simulink model "PathNavHardwareV2"  (R2021a)
settings: Solver=FixedStepAuto  StartTime=0.0  StopTime=10.0  RelTol=1e-3
values from neighbouring files (symbols this model uses):
  axleLength = 0.136    [robotParameters.m]
  ticksPerRot = 20    [robotParameters.m]
  wheelR = 0.031    [robotParameters.m]
undefined symbols (not defined in the file or in its folder): InputPWM, WheelSpeed
libraries: arduinolib x11, pid_lib x5, spsEdgeDetectorLib x2, simulink_extras x1, mobileRoboticsTrainingLib x1
settings Model: SILPILModeSetting=veronly  ExtModeTrigDuration=2  Creator=Marc  LastModifiedBy=Marc
settings OptimizationCC: EnhancedBackFolding=on  PassReuseOutputArgsAs=Individual arguments  ZeroExternalMemoryAtStartup=off  ZeroInternalMemoryAtStartup=off  MaxStackSize=64  OptimizeBlockOrder=speed  DifferentSizesBufferReuse=on  OptimizationCustomize=off  EfficientTunableParamExpr=on
settings DebuggingCC: ParameterTunabilityLossMsg=error
settings HardwareCC: ProdBitPerInt=16  ProdBitPerPointer=16  ProdBitPerSizeT=16  ProdBitPerPtrDiffT=16  ProdLargestAtomicFloat=None  ProdWordSize=8  ProdHWDeviceType=Atmel->AVR  UseEmbeddedCoderFeatures=off  UseSimulinkCoderFeatures=off
settings SFSimCC: MATLABDynamicMemAlloc=off
settings RTWCC: SystemTargetFile=ert.tlc  HardwareBoard=Arduino Leonardo  TemplateMakefile=ert_default_tmf  Toolchain=Arduino AVR
settings CodeAppCC: ForceParamTrailComments=on  IgnoreCustomStorageClasses=off  OperatorAnnotations=on  SimulinkDataObjDesc=on  SFDataObjDesc=on  InsertBlockDesc=on
settings ERTTargetCC: SupportContinuousTime=on  SupportNonInlinedSFcns=on  SupportVariableSizeSignals=on  ExtModeTransport=5  ExtModeStaticAllocSize=250  ExtModeMexFile=ext_serial_win32_comm_leonardo

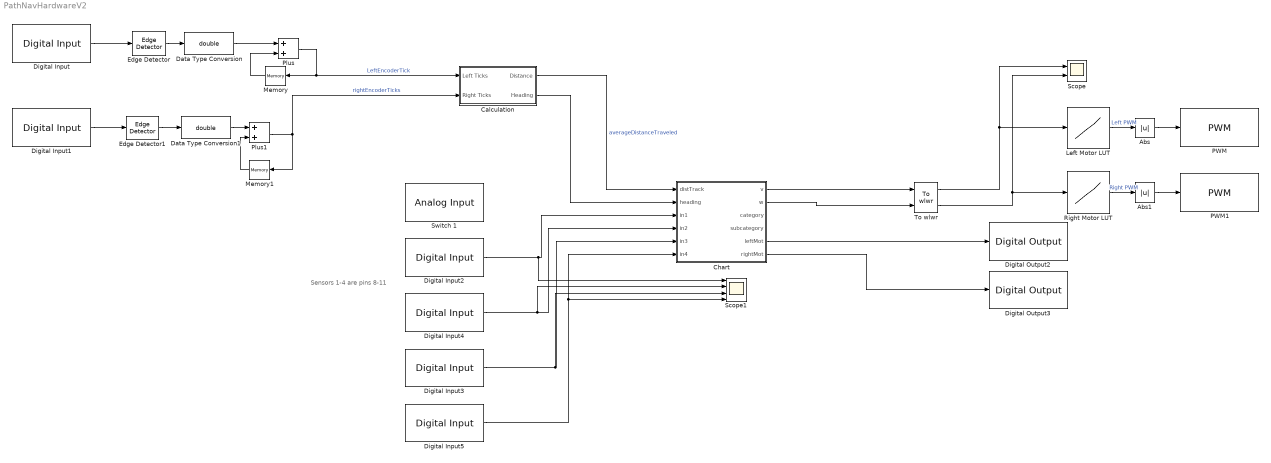
== system PathNavHardwareV2 ==
  note: Sensors 1-4 are pins 8-11
  Abs : Abs
  Abs1 : Abs
  Calculation : Subsystem
  Chart : Stateflow chart  TreatAsAtomicUnit=on
  Data Type Conversion : DataTypeConversion  OutDataTypeStr=double
  Data Type Conversion1 : DataTypeConversion  OutDataTypeStr=double
  Digital Input : arduinolib/Digital Input  pinNumber=2  mode=Default  Direction=input  SampleTime=0.01  blockPlatform=arduino
  Digital Input1 : arduinolib/Digital Input  pinNumber=3  mode=Default  Direction=input  SampleTime=0.01  blockPlatform=arduino
  Digital Input2 : arduinolib/Digital Input  pinNumber=8  mode=Default  Direction=input  SampleTime=0.01  blockPlatform=arduino
  Digital Input3 : arduinolib/Digital Input  pinNumber=10  mode=Default  Direction=input  SampleTime=0.01  blockPlatform=arduino
  Digital Input4 : arduinolib/Digital Input  pinNumber=9  mode=Default  Direction=input  SampleTime=0.01  blockPlatform=arduino
  Digital Input5 : arduinolib/Digital Input  pinNumber=11  mode=Default  Direction=input  SampleTime=0.01  blockPlatform=arduino
  Digital Output2 : arduinolib/Digital Output  pinNumber=4  Direction=output  blockPlatform=arduino
  Digital Output3 : arduinolib/Digital Output  pinNumber=7  Direction=output  blockPlatform=arduino
  Edge Detector : spsEdgeDetectorLib/Edge Detector  model=Either  ic=0  Ts=0
      settings: SourceProductBaseCode=PS
  Edge Detector1 : spsEdgeDetectorLib/Edge Detector  model=Either  ic=0  Ts=0
      settings: SourceProductBaseCode=PS
  Left Motor LUT : Lookup_n-D  NumberOfTableDimensions=1  BreakpointsForDimension1=WheelSpeed  Table=InputPWM  InterpMethod=Nearest  ExtrapMethod=Clip  InternalRulePriority=Speed  RndMeth=Simplest  InputSameDT=on
  Memory : Memory
  Memory1 : Memory
  PWM : arduinolib/PWM  pinNumber=5  frequencyType=Default  desiredFrequency=490.2  achievableFrequency=490.2
  PWM1 : arduinolib/PWM  pinNumber=6  frequencyType=Default  desiredFrequency=490.2  achievableFrequency=490.2
  Plus : Sum
  Plus1 : Sum
  Right Motor LUT : Lookup_n-D  NumberOfTableDimensions=1  BreakpointsForDimension1=WheelSpeed  Table=InputPWM  InterpMethod=Nearest  ExtrapMethod=Clip  InternalRulePriority=Speed  RndMeth=Simplest  InputSameDT=on
  Scope : Scope  NumInputPorts=2
  Scope1 : Scope  NumInputPorts=4
  Switch 1 : arduinolib/Analog Input  pinNumber=0  ReadResultsOnly=off  ConversionTriggerSource=Software  ExternalTriggerType=uint32( 0 )  OutputDataType=uint16  EnableConversionCompleteNotify=off  EnableOuputStatus=off  SampleTime=0.01  blockPlatform=arduino
  To wlwr : mobileRoboticsTrainingLib/To wlwr  axleLength=0.1  wheelR=0.05
  wires:
  Edge Detector1/1 -> Data Type Conversion1/1
  Edge Detector/1 -> Data Type Conversion/1
  Plus1/1 -> Calculation/2(Right Ticks), Memory1/1  "rightEncoderTicks"
  To wlwr/1 -> Scope/1, Left Motor LUT/1
  Digital Input1/1 -> Edge Detector1/1
  Left Motor LUT/1 -> Abs/1  "Left PWM"
  Data Type Conversion/1 -> Plus/1
  Plus/1 -> Calculation/1(Left Ticks), Memory/1  "LeftEncoderTick"
  Digital Input/1 -> Edge Detector/1
  Memory/1 -> Plus/2
  Memory1/1 -> Plus1/2
  Data Type Conversion1/1 -> Plus1/1
  Right Motor LUT/1 -> Abs1/1  "Right PWM"
  To wlwr/2 -> Scope/2, Right Motor LUT/1
  Calculation/1(Distance) -> Chart/1(distTrack)  "averageDistanceTraveled"
  Calculation/2(Heading) -> Chart/2(heading)
  Digital Input2/1 -> Scope1/1, Chart/3(in1)
  Digital Input4/1 -> Scope1/2, Chart/4(in2)
  Digital Input3/1 -> Chart/5(in3), Scope1/3
  Digital Input5/1 -> Scope1/4, Chart/6(in4)
  Chart/1(v) -> To wlwr/1
  Chart/2(w) -> To wlwr/2
  Chart/5(leftMot) -> Digital Output2/1
  Chart/6(rightMot) -> Digital Output3/1
  Abs/1 -> PWM/1
  Abs1/1 -> PWM1/1

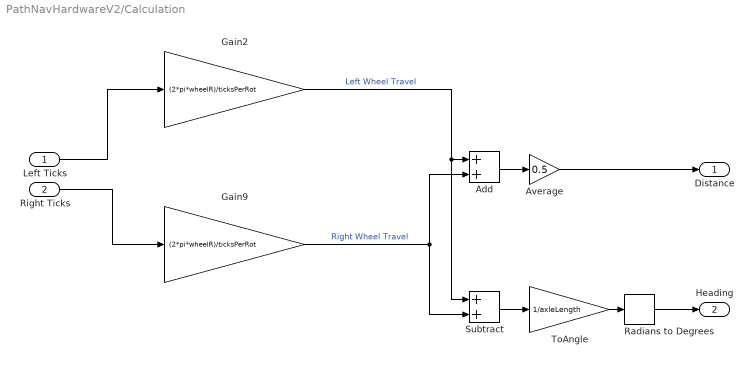
== system PathNavHardwareV2/Calculation ==
  Left Ticks : Inport
  Right Ticks : Inport  Port=2
  Add : Sum
  Average : Gain  Gain=0.5
  Gain2 : Gain  Gain=(2*pi*wheelR)/ticksPerRot
  Gain9 : Gain  Gain=(2*pi*wheelR)/ticksPerRot
  Radians to Degrees : simulink_extras/Transformations/Radians to Degrees
  Subtract : Sum
  ToAngle : Gain  Gain=1/axleLength
  Distance : Outport
  Heading : Outport  Port=2
  wires:
  Average/1 -> Distance/1
  Add/1 -> Average/1
  Gain2/1 -> Subtract/1, Add/1  "Left Wheel Travel"
  Right Ticks/1 -> Gain9/1
  Left Ticks/1 -> Gain2/1
  Gain9/1 -> Subtract/2, Add/2  "Right Wheel Travel"
  Subtract/1 -> ToAngle/1
  ToAngle/1 -> Radians to Degrees/1
  Radians to Degrees/1 -> Heading/1

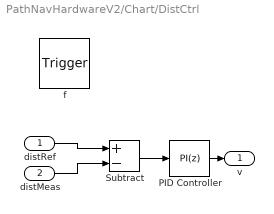
== system PathNavHardwareV2/Chart/DistCtrl ==
  distRef : Inport  OutDataTypeStr=double  PortDimensions=1
  distMeas : Inport  Port=2  OutDataTypeStr=double  PortDimensions=1
  f : TriggerPort  TriggerType=function-call  VariantControl=Variant
      settings: CopyFcn=Stateflow.SLINSF.SimulinkMan.removeBlockPreDeleteFcn  PreDeleteFcn=Stateflow.SLINSF.SimulinkMan.unsafePredeleteFcn
  PID Controller : pid_lib/PID Controller  Controller=PI  Form=Parallel  TimeDomain=Discrete-time  UseExternalTs=off  SampleTime=-1  IntegratorMethod=Forward Euler  FilterMethod=Forward Euler  ControllerParametersSource=internal  P=1.1  I=0.2  D=-0.0140783779685636  UseFilter=off  N=151.701833251505  TunerSelectOption=Transfer Function Based (PID Tuner App)  InitialConditionSource=internal  InitialConditionForIntegrator=0  InitialConditionForFilter=0  DifferentiatorICPrevScaledInput=0  ExternalReset=none  TrackingMode=off  Kt=1  LimitOutput=on  SatLimitsSource=internal  UpperSaturationLimit=0.6  LowerSaturationLimit=-0.6  LinearizeAsGain=on  AntiWindupMode=clamping  Kb=1  POutMin=[]  POutMax=[]  IOutMin=[]  IOutMax=[]  DOutMin=[]  DOutMax=[]  NOutMin=[]  NOutMax=[]  SumOutMin=[]  SumOutMax=[]  SaturationOutMin=[]  SaturationOutMax=[]  PParamMin=[]  PParamMax=[]  IParamMin=[]  IParamMax=[]  DParamMin=[]  DParamMax=[]  NParamMin=[]  NParamMax=[]  KbParamMin=[]  KbParamMax=[]  KtParamMin=[]  KtParamMax=[]  KbOutMin=[]  KbOutMax=[]  KtOutMin=[]  KtOutMax=[]  IntegratorOutMin=[]  IntegratorOutMax=[]  FilterOutMin=[]  FilterOutMax=[]  SumI1OutMin=[]  SumI1OutMax=[]  SumI2OutMin=[]  SumI2OutMax=[]  SumI3OutMin=[]  SumI3OutMax=[]  SumI4OutMin=[]  SumI4OutMax=[]  SumDOutMin=[]  SumDOutMax=[]  DifferentiatorOutMin=[]  DifferentiatorOutMax=[]  FilterDiffOutCoefMin=[]  FilterDiffOutCoefMax=[]  ReciprocalOutMin=[]  ReciprocalOutMax=[]  SumDenOutMin=[]  SumDenOutMax=[]  SumNumOutMin=[]  SumNumOutMax=[]  DivideOutMin=[]  DivideOutMax=[]  UdiffTsProdOutMin=[]  UdiffTsProdOutMax=[]  NTsProdOutMin=[]  NTsProdOutMax=[]  UintegralTsProdOutMin=[]  UintegralTsProdOutMax=[]  UngainTsProdOutMin=[]  UngainTsProdOutMax=[]  IntegratorContinuousStateAttributes=''  IntegratorStateMustResolveToSignalObject=off  IntegratorRTWStateStorageClass=Auto  FilterContinuousStateAttributes=''  FilterStateMustResolveToSignalObject=off  FilterRTWStateStorageClass=Auto  ParallelPVariant=InternalParameters  IdealPVariant=Disabled  IVariant=InternalParameters  DVariant=Disabled  IntegratorVariant=Discrete  SatVariant=Enabled  AWVariant=DiscClampingParallel  PCopyVariant=Disabled  TRVariant=Disabled  FdbkBlocksVariant=Forward  IdealPFdbkVariant=Disabled  SatFdbkVariant=Disabled  DerivativeFilterVariant=Disabled  NVariant=Disabled  NCopyVariant=Disabled_SignalSpec  FilterICVariant=Disabled  IntegratorICVariant=InternalICs  ExternalResetVariant=Disabled  TRSumVariant=Passthrough  SumFdbkVariant=Disabled  SumVariant=Sum_PI  TsampFilterVariant=InternalTs  TsampNgainVariant=Passthrough  TsampIntegralVariant=Passthrough  ExternalSaturationOutDataTypeStr=Inherit: Same as second input  InitialConditionSetting=Output
  Subtract : Sum  Inputs=+-
  v : Outport
  wires:
  Subtract/1 -> PID Controller/1
  PID Controller/1 -> v/1
  distRef/1 -> Subtract/1
  distMeas/1 -> Subtract/2

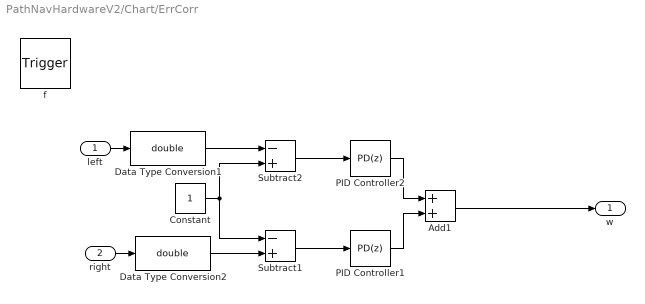
== system PathNavHardwareV2/Chart/ErrCorr ==
  left : Inport  OutDataTypeStr=double  PortDimensions=1
  right : Inport  Port=2  OutDataTypeStr=double  PortDimensions=1
  f : TriggerPort  TriggerType=function-call  VariantControl=(inherit)
      settings: CopyFcn=Stateflow.SLINSF.SimulinkMan.removeBlockPreDeleteFcn  PreDeleteFcn=Stateflow.SLINSF.SimulinkMan.unsafePredeleteFcn
  Add1 : Sum
  Constant : Constant
  Data Type Conversion1 : DataTypeConversion  OutDataTypeStr=double
  Data Type Conversion2 : DataTypeConversion  OutDataTypeStr=double
  PID Controller1 : pid_lib/PID Controller  Controller=PD  Form=Parallel  TimeDomain=Discrete-time  UseExternalTs=off  SampleTime=-1  IntegratorMethod=Forward Euler  FilterMethod=Forward Euler  ControllerParametersSource=internal  P=1.5  I=1  D=1e-5  UseFilter=on  N=100  TunerSelectOption=Transfer Function Based (PID Tuner App)  InitialConditionSource=internal  InitialConditionForIntegrator=0  InitialConditionForFilter=0  DifferentiatorICPrevScaledInput=0  ExternalReset=none  TrackingMode=off  Kt=1  LimitOutput=off  SatLimitsSource=internal  UpperSaturationLimit=inf  LowerSaturationLimit=-inf  LinearizeAsGain=on  AntiWindupMode=none  Kb=1  POutMin=[]  POutMax=[]  IOutMin=[]  IOutMax=[]  DOutMin=[]  DOutMax=[]  NOutMin=[]  NOutMax=[]  SumOutMin=[]  SumOutMax=[]  SaturationOutMin=[]  SaturationOutMax=[]  PParamMin=[]  PParamMax=[]  IParamMin=[]  IParamMax=[]  DParamMin=[]  DParamMax=[]  NParamMin=[]  NParamMax=[]  KbParamMin=[]  KbParamMax=[]  KtParamMin=[]  KtParamMax=[]  KbOutMin=[]  KbOutMax=[]  KtOutMin=[]  KtOutMax=[]  IntegratorOutMin=[]  IntegratorOutMax=[]  FilterOutMin=[]  FilterOutMax=[]  SumI1OutMin=[]  SumI1OutMax=[]  SumI2OutMin=[]  SumI2OutMax=[]  SumI3OutMin=[]  SumI3OutMax=[]  SumI4OutMin=[]  SumI4OutMax=[]  SumDOutMin=[]  SumDOutMax=[]  DifferentiatorOutMin=[]  DifferentiatorOutMax=[]  FilterDiffOutCoefMin=[]  FilterDiffOutCoefMax=[]  ReciprocalOutMin=[]  ReciprocalOutMax=[]  SumDenOutMin=[]  SumDenOutMax=[]  SumNumOutMin=[]  SumNumOutMax=[]  DivideOutMin=[]  DivideOutMax=[]  UdiffTsProdOutMin=[]  UdiffTsProdOutMax=[]  NTsProdOutMin=[]  NTsProdOutMax=[]  UintegralTsProdOutMin=[]  UintegralTsProdOutMax=[]  UngainTsProdOutMin=[]  UngainTsProdOutMax=[]  IntegratorContinuousStateAttributes=''  IntegratorStateMustResolveToSignalObject=off  IntegratorRTWStateStorageClass=Auto  FilterContinuousStateAttributes=''  FilterStateMustResolveToSignalObject=off  FilterRTWStateStorageClass=Auto  ParallelPVariant=InternalParameters  IdealPVariant=Disabled  IVariant=Disabled  DVariant=InternalParameters  IntegratorVariant=Disabled  SatVariant=Disabled  AWVariant=Disabled  PCopyVariant=Disabled  TRVariant=Disabled  FdbkBlocksVariant=Forward  IdealPFdbkVariant=Disabled  SatFdbkVariant=Disabled  DerivativeFilterVariant=ForwardEulerFilter  NVariant=InternalParameters  NCopyVariant=Disabled  FilterICVariant=InternalICsFilter  IntegratorICVariant=Disabled  ExternalResetVariant=Disabled  TRSumVariant=Passthrough  SumFdbkVariant=Disabled  SumVariant=Sum_PD  TsampFilterVariant=InternalTs  TsampNgainVariant=Passthrough  TsampIntegralVariant=Disabled_SignalSpec  ExternalSaturationOutDataTypeStr=Inherit: Same as second input  InitialConditionSetting=Output
  PID Controller2 : pid_lib/PID Controller  Controller=PD  Form=Parallel  TimeDomain=Discrete-time  UseExternalTs=off  SampleTime=-1  IntegratorMethod=Forward Euler  FilterMethod=Forward Euler  ControllerParametersSource=internal  P=1.5  I=1  D=1e-5  UseFilter=on  N=100  TunerSelectOption=Transfer Function Based (PID Tuner App)  InitialConditionSource=internal  InitialConditionForIntegrator=0  InitialConditionForFilter=0  DifferentiatorICPrevScaledInput=0  ExternalReset=none  TrackingMode=off  Kt=1  LimitOutput=off  SatLimitsSource=internal  UpperSaturationLimit=inf  LowerSaturationLimit=-inf  LinearizeAsGain=on  AntiWindupMode=none  Kb=1  POutMin=[]  POutMax=[]  IOutMin=[]  IOutMax=[]  DOutMin=[]  DOutMax=[]  NOutMin=[]  NOutMax=[]  SumOutMin=[]  SumOutMax=[]  SaturationOutMin=[]  SaturationOutMax=[]  PParamMin=[]  PParamMax=[]  IParamMin=[]  IParamMax=[]  DParamMin=[]  DParamMax=[]  NParamMin=[]  NParamMax=[]  KbParamMin=[]  KbParamMax=[]  KtParamMin=[]  KtParamMax=[]  KbOutMin=[]  KbOutMax=[]  KtOutMin=[]  KtOutMax=[]  IntegratorOutMin=[]  IntegratorOutMax=[]  FilterOutMin=[]  FilterOutMax=[]  SumI1OutMin=[]  SumI1OutMax=[]  SumI2OutMin=[]  SumI2OutMax=[]  SumI3OutMin=[]  SumI3OutMax=[]  SumI4OutMin=[]  SumI4OutMax=[]  SumDOutMin=[]  SumDOutMax=[]  DifferentiatorOutMin=[]  DifferentiatorOutMax=[]  FilterDiffOutCoefMin=[]  FilterDiffOutCoefMax=[]  ReciprocalOutMin=[]  ReciprocalOutMax=[]  SumDenOutMin=[]  SumDenOutMax=[]  SumNumOutMin=[]  SumNumOutMax=[]  DivideOutMin=[]  DivideOutMax=[]  UdiffTsProdOutMin=[]  UdiffTsProdOutMax=[]  NTsProdOutMin=[]  NTsProdOutMax=[]  UintegralTsProdOutMin=[]  UintegralTsProdOutMax=[]  UngainTsProdOutMin=[]  UngainTsProdOutMax=[]  IntegratorContinuousStateAttributes=''  IntegratorStateMustResolveToSignalObject=off  IntegratorRTWStateStorageClass=Auto  FilterContinuousStateAttributes=''  FilterStateMustResolveToSignalObject=off  FilterRTWStateStorageClass=Auto  ParallelPVariant=InternalParameters  IdealPVariant=Disabled  IVariant=Disabled  DVariant=InternalParameters  IntegratorVariant=Disabled  SatVariant=Disabled  AWVariant=Disabled  PCopyVariant=Disabled  TRVariant=Disabled  FdbkBlocksVariant=Forward  IdealPFdbkVariant=Disabled  SatFdbkVariant=Disabled  DerivativeFilterVariant=ForwardEulerFilter  NVariant=InternalParameters  NCopyVariant=Disabled  FilterICVariant=InternalICsFilter  IntegratorICVariant=Disabled  ExternalResetVariant=Disabled  TRSumVariant=Passthrough  SumFdbkVariant=Disabled  SumVariant=Sum_PD  TsampFilterVariant=InternalTs  TsampNgainVariant=Passthrough  TsampIntegralVariant=Disabled_SignalSpec  ExternalSaturationOutDataTypeStr=Inherit: Same as second input  InitialConditionSetting=Output
  Subtract1 : Sum  Inputs=-+
  Subtract2 : Sum  Inputs=-+
  w : Outport
  wires:
  Subtract2/1 -> PID Controller2/1
  Subtract1/1 -> PID Controller1/1
  PID Controller1/1 -> Add1/2
  Constant/1 -> Subtract2/2, Subtract1/1
  left/1 -> Data Type Conversion1/1
  right/1 -> Data Type Conversion2/1
  PID Controller2/1 -> Add1/1
  Data Type Conversion2/1 -> Subtract1/2
  Data Type Conversion1/1 -> Subtract2/1
  Add1/1 -> w/1

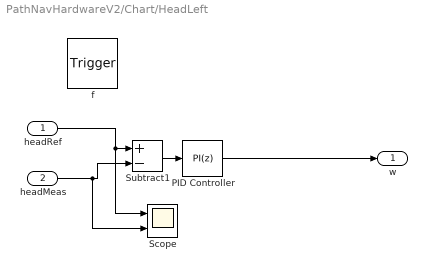
== system PathNavHardwareV2/Chart/HeadLeft ==
  headRef : Inport  OutDataTypeStr=double  PortDimensions=1
  headMeas : Inport  Port=2  OutDataTypeStr=double  PortDimensions=1
  f : TriggerPort  TriggerType=function-call  VariantControl=(inherit)
      settings: CopyFcn=Stateflow.SLINSF.SimulinkMan.removeBlockPreDeleteFcn  PreDeleteFcn=Stateflow.SLINSF.SimulinkMan.unsafePredeleteFcn
  PID Controller : pid_lib/PID Controller  Controller=PI  Form=Parallel  TimeDomain=Discrete-time  UseExternalTs=off  SampleTime=-1  IntegratorMethod=Forward Euler  FilterMethod=Forward Euler  ControllerParametersSource=internal  P=0.1  I=0.001  D=-0.0140783779685636  UseFilter=off  N=151.701833251505  TunerSelectOption=Transfer Function Based (PID Tuner App)  InitialConditionSource=internal  InitialConditionForIntegrator=0  InitialConditionForFilter=0  DifferentiatorICPrevScaledInput=0  ExternalReset=none  TrackingMode=off  Kt=1  LimitOutput=on  SatLimitsSource=internal  UpperSaturationLimit=4  LowerSaturationLimit=-4  LinearizeAsGain=on  AntiWindupMode=clamping  Kb=1  POutMin=[]  POutMax=[]  IOutMin=[]  IOutMax=[]  DOutMin=[]  DOutMax=[]  NOutMin=[]  NOutMax=[]  SumOutMin=[]  SumOutMax=[]  SaturationOutMin=[]  SaturationOutMax=[]  PParamMin=[]  PParamMax=[]  IParamMin=[]  IParamMax=[]  DParamMin=[]  DParamMax=[]  NParamMin=[]  NParamMax=[]  KbParamMin=[]  KbParamMax=[]  KtParamMin=[]  KtParamMax=[]  KbOutMin=[]  KbOutMax=[]  KtOutMin=[]  KtOutMax=[]  IntegratorOutMin=[]  IntegratorOutMax=[]  FilterOutMin=[]  FilterOutMax=[]  SumI1OutMin=[]  SumI1OutMax=[]  SumI2OutMin=[]  SumI2OutMax=[]  SumI3OutMin=[]  SumI3OutMax=[]  SumI4OutMin=[]  SumI4OutMax=[]  SumDOutMin=[]  SumDOutMax=[]  DifferentiatorOutMin=[]  DifferentiatorOutMax=[]  FilterDiffOutCoefMin=[]  FilterDiffOutCoefMax=[]  ReciprocalOutMin=[]  ReciprocalOutMax=[]  SumDenOutMin=[]  SumDenOutMax=[]  SumNumOutMin=[]  SumNumOutMax=[]  DivideOutMin=[]  DivideOutMax=[]  UdiffTsProdOutMin=[]  UdiffTsProdOutMax=[]  NTsProdOutMin=[]  NTsProdOutMax=[]  UintegralTsProdOutMin=[]  UintegralTsProdOutMax=[]  UngainTsProdOutMin=[]  UngainTsProdOutMax=[]  IntegratorContinuousStateAttributes=''  IntegratorStateMustResolveToSignalObject=off  IntegratorRTWStateStorageClass=Auto  FilterContinuousStateAttributes=''  FilterStateMustResolveToSignalObject=off  FilterRTWStateStorageClass=Auto  ParallelPVariant=InternalParameters  IdealPVariant=Disabled  IVariant=InternalParameters  DVariant=Disabled  IntegratorVariant=Discrete  SatVariant=Enabled  AWVariant=DiscClampingParallel  PCopyVariant=Disabled  TRVariant=Disabled  FdbkBlocksVariant=Forward  IdealPFdbkVariant=Disabled  SatFdbkVariant=Disabled  DerivativeFilterVariant=Disabled  NVariant=Disabled  NCopyVariant=Disabled_SignalSpec  FilterICVariant=Disabled  IntegratorICVariant=InternalICs  ExternalResetVariant=Disabled  TRSumVariant=Passthrough  SumFdbkVariant=Disabled  SumVariant=Sum_PI  TsampFilterVariant=InternalTs  TsampNgainVariant=Passthrough  TsampIntegralVariant=Passthrough  ExternalSaturationOutDataTypeStr=Inherit: Same as second input  InitialConditionSetting=Output
  Scope : Scope  NumInputPorts=2
  Subtract1 : Sum  Inputs=+-
  w : Outport
  wires:
  Subtract1/1 -> PID Controller/1
  headMeas/1 -> Scope/2, Subtract1/2
  headRef/1 -> Scope/1, Subtract1/1
  PID Controller/1 -> w/1

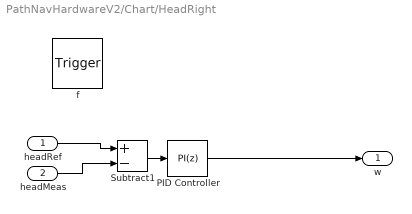
== system PathNavHardwareV2/Chart/HeadRight ==
  headRef : Inport  OutDataTypeStr=double  PortDimensions=1
  headMeas : Inport  Port=2  OutDataTypeStr=double  PortDimensions=1
  f : TriggerPort  TriggerType=function-call  VariantControl=(inherit)
      settings: CopyFcn=Stateflow.SLINSF.SimulinkMan.removeBlockPreDeleteFcn  PreDeleteFcn=Stateflow.SLINSF.SimulinkMan.unsafePredeleteFcn
  PID Controller : pid_lib/PID Controller  Controller=PI  Form=Parallel  TimeDomain=Discrete-time  UseExternalTs=off  SampleTime=-1  IntegratorMethod=Forward Euler  FilterMethod=Forward Euler  ControllerParametersSource=internal  P=0.1  I=0.001  D=-0.0140783779685636  UseFilter=off  N=151.701833251505  TunerSelectOption=Transfer Function Based (PID Tuner App)  InitialConditionSource=internal  InitialConditionForIntegrator=0  InitialConditionForFilter=0  DifferentiatorICPrevScaledInput=0  ExternalReset=none  TrackingMode=off  Kt=1  LimitOutput=on  SatLimitsSource=internal  UpperSaturationLimit=4  LowerSaturationLimit=-4  LinearizeAsGain=on  AntiWindupMode=clamping  Kb=1  POutMin=[]  POutMax=[]  IOutMin=[]  IOutMax=[]  DOutMin=[]  DOutMax=[]  NOutMin=[]  NOutMax=[]  SumOutMin=[]  SumOutMax=[]  SaturationOutMin=[]  SaturationOutMax=[]  PParamMin=[]  PParamMax=[]  IParamMin=[]  IParamMax=[]  DParamMin=[]  DParamMax=[]  NParamMin=[]  NParamMax=[]  KbParamMin=[]  KbParamMax=[]  KtParamMin=[]  KtParamMax=[]  KbOutMin=[]  KbOutMax=[]  KtOutMin=[]  KtOutMax=[]  IntegratorOutMin=[]  IntegratorOutMax=[]  FilterOutMin=[]  FilterOutMax=[]  SumI1OutMin=[]  SumI1OutMax=[]  SumI2OutMin=[]  SumI2OutMax=[]  SumI3OutMin=[]  SumI3OutMax=[]  SumI4OutMin=[]  SumI4OutMax=[]  SumDOutMin=[]  SumDOutMax=[]  DifferentiatorOutMin=[]  DifferentiatorOutMax=[]  FilterDiffOutCoefMin=[]  FilterDiffOutCoefMax=[]  ReciprocalOutMin=[]  ReciprocalOutMax=[]  SumDenOutMin=[]  SumDenOutMax=[]  SumNumOutMin=[]  SumNumOutMax=[]  DivideOutMin=[]  DivideOutMax=[]  UdiffTsProdOutMin=[]  UdiffTsProdOutMax=[]  NTsProdOutMin=[]  NTsProdOutMax=[]  UintegralTsProdOutMin=[]  UintegralTsProdOutMax=[]  UngainTsProdOutMin=[]  UngainTsProdOutMax=[]  IntegratorContinuousStateAttributes=''  IntegratorStateMustResolveToSignalObject=off  IntegratorRTWStateStorageClass=Auto  FilterContinuousStateAttributes=''  FilterStateMustResolveToSignalObject=off  FilterRTWStateStorageClass=Auto  ParallelPVariant=InternalParameters  IdealPVariant=Disabled  IVariant=InternalParameters  DVariant=Disabled  IntegratorVariant=Discrete  SatVariant=Enabled  AWVariant=DiscClampingParallel  PCopyVariant=Disabled  TRVariant=Disabled  FdbkBlocksVariant=Forward  IdealPFdbkVariant=Disabled  SatFdbkVariant=Disabled  DerivativeFilterVariant=Disabled  NVariant=Disabled  NCopyVariant=Disabled_SignalSpec  FilterICVariant=Disabled  IntegratorICVariant=InternalICs  ExternalResetVariant=Disabled  TRSumVariant=Passthrough  SumFdbkVariant=Disabled  SumVariant=Sum_PI  TsampFilterVariant=InternalTs  TsampNgainVariant=Passthrough  TsampIntegralVariant=Passthrough  ExternalSaturationOutDataTypeStr=Inherit: Same as second input  InitialConditionSetting=Output
  Subtract1 : Sum  Inputs=+-
  w : Outport
  wires:
  Subtract1/1 -> PID Controller/1
  headMeas/1 -> Subtract1/2
  headRef/1 -> Subtract1/1
  PID Controller/1 -> w/1

== stateflow chart PathNavHardwareV2/Chart ==
  state LineFollow
    entry:
    leftMot=0;
    rightMot=0;
    state EndOfMaze
      entry:
      v=0;
      w=0;
      subcategory= 1;
    state CrossRoads
      entry:
      v=0;
      w=0;
      subcategory= 2;
    state Junction1_0000_
      entry:
      v=0.1;
      w=0;
      stopDist=0.018
      startDist = distTrack
      category = 2
    state MoveForward
      entry:
      v=0.1;
      stopDist=2
      category = 1
      during:
      w=ErrCorr(in2,in3);
    state J0000
      entry:
      v=0
    state TJunc
      entry:
      v=0;
      w=0;
      subcategory= 3;
    state Initial
      entry:
      v=0;
      w=0;
      stopDist=0;
      category= 0;
    state StartDetect
      entry,during:
      stopDist=0
      %w=ErrCorr(in2,in3);
    state Junction2_1000_
      entry:
      v=0.1;
      w=0;
      stopDist=0.018
      startDist = distTrack
      category = 3
    state RightTurn
      entry:
      v=0;
      w=0;
      subcategory= 1;
    state J1000
      entry:
      v=0
    state RightTJunc
      entry:
      v=0;
      w=0;
      subcategory= 2;
    state Junction3_0001_
      entry:
      v=0.1;
      w=0;
      stopDist=0.018
      startDist = distTrack
      category = 4
    state J0001
      entry:
      v=0
    state LeftTurn
      entry:
      v=0;
      w=0;
      subcategory= 1;
    state DeadEnd1
    state LeftTJunc
      entry:
      v=0;
      w=0;
      subcategory= 2;
    state DeadEnd
      entry:
      v=0;
      w=0;
      category = 5
      subcategory= 1;
    Junction1_0000_ -> EndOfMaze [order 1] : [distTrack >= (startDist + 0.075) & in1==0 & in2==0 & in3==0 & in4==0 ]
    Junction1_0000_ -> CrossRoads [order 2] : [distTrack >= (startDist +0.05) & in1==1 & in2==0 & in3==0 & in4==1 ]
    (default) -> Initial
    MoveForward -> J0000 [order 1] : [in1==0 & in2==0 & in3==0 & in4==0]
    Junction1_0000_ -> TJunc [order 3] : [distTrack >= (startDist + 0.05) & in1==1 & in2==1 & in3==1 & in4==1 ]
    J0000 -> MoveForward [order 2] : [in1==1 || in4==1]
    J0000 -> Junction1_0000_ [order 1] : after(0.01,sec) [in1==0 & in2==0 & in3==0 & in4==0]
    StartDetect -> MoveForward : [in2==0 & in3==0]
    Initial -> StartDetect
    Junction2_1000_ -> RightTurn [order 1] : [distTrack >= (startDist + 0.059) & in1==1 & in2==1 & in3==1 & in4==1 ]
    MoveForward -> J1000 [order 2] : [in1==1 & in2==0 & in3==0 & in4==0]
    J1000 -> MoveForward [order 2] : [in1==0 || in4==1]
    Junction2_1000_ -> RightTJunc [order 2] : [distTrack >= (startDist + 0.01) & in1==1 & in2==0 & in3==0 & in4==1 ]
    J1000 -> Junction2_1000_ [order 1] : after(0.05,sec) [in1==1 & in2==0 & in3==0 & in4==0]
    DeadEnd1 -> MoveForward [order 1] : [in1==0 || in2==0 || in3==0 || in4==0]
    MoveForward -> DeadEnd1 [order 4] : [in1==1 & in2==1 & in3==1 & in4==1]
    J0001 -> MoveForward [order 2] : [in1==1 || in4==0]
    MoveForward -> J0001 [order 3] : [in1==0 & in2==0 & in3==0 & in4==1]
    J0001 -> Junction3_0001_ [order 1] : after(0.01, sec) [in1==0 & in2==0 & in3==0 & in4==1]
    Junction3_0001_ -> LeftTurn [order 1] : [distTrack >= (startDist + 0.05) & in1==1 & in2==1 & in3==1 & in4==1]
    Junction3_0001_ -> LeftTJunc [order 2] : [distTrack >= (startDist + 0.05) & in1==1 & in2==0 & in3==0 & in4==1 ]
    DeadEnd1 -> DeadEnd [order 2] : after(0.05,sec) [in1==1 & in2==1 & in3==1 & in4==1]
  state Left
    state Rotate
      entry:
      currHead=heading
      v=0;
      leftMot=5;
      rightMot=0;
      during:
      w=HeadLeft(95+currHead,heading);
    state Stop
      entry:
      w=0
      currHead=heading
    (default) -> Left.Rotate
    Left.Rotate -> Left.Stop : [heading-currHead>=95]{currHead=heading}
  state w=HeadLeft(headRef,headMeas) [function]
  state v = DistCtrl(distRef,distMeas) [function]
  state w=ErrCorr(left,right) [function]
  state Straight
  state w=HeadRight(headRef,headMeas) [function]
  state Right
    state Rotate
      entry:
      currHead=heading
      during:
      w=HeadRight(currHead-90,heading);
    state Stop
      entry:
      w=0
      currHead=heading
    (default) -> Right.Rotate
    Right.Rotate -> Right.Stop : [heading-currHead<=-90]{currHead=heading}
  state Back
    state Rotate
      entry:
      currHead=heading
      v=0;
      leftMot=5;
      rightMot=0;
      during:
      w=HeadLeft(180+currHead,heading);
    state Stop
      entry:
      w=0
    (default) -> Back.Rotate
    Back.Rotate -> Back.Stop : [heading-currHead>=180]{currHead=heading}
  Left.Stop -> LineFollow : after(0.25,sec)
  (default) -> LineFollow
  CrossRoads -> Left
  TJunc -> Left
  LeftTurn -> Left
  LeftTJunc -> Left
  RightTurn -> Right
  RightTJunc -> Straight
  Straight -> LineFollow
  Right.Stop -> LineFollow
  DeadEnd -> Back
  Back.Stop -> LineFollow
  data: headRef function_input double size=1; headMeas function_input double size=1; w function_output; distRef function_input double size=1; distMeas function_input double size=1; v function_output; left function_input double size=1; right function_input double size=1; w function_output; headRef function_input double size=1; headMeas function_input double size=1; w function_output; distTrack input; heading input; in1 input; in2 input; in3 input; in4 input; v output; w output; category output; subcategory output; startDist local; stopDist local; currHead local; leftMot output; rightMot output
